simulink model "wlan_mac_hw"  (Simulink 7.8)
settings: Solver=ode45  StartTime=0.0  StopTime=200  RelTol=1e-3
PostLoadFcn:
  | wlan_mac_hw_init
InitFcn:
  | wlan_mac_hw_init
StartFcn:
  | wlan_mac_hw_init
values from neighbouring files (symbols this model uses):
  NB_CNTR_NAV = ceil(log2(MAX_NAV * 160))    [wlan_mac_hw_init.m]
  ticks_per_usec = 10    [wlan_mac_hw_init.m]
undefined symbols (not defined in the file or in its folder): gcbh, xlBlockLoadCallback, xlGetNormalizedPeriod
libraries: xbsIndex_r4 x788, xbsEDKLib_r4 x1
(part 3 of 6)

== system wlan_mac_hw/Idle for DIFS-EIFS ==
  note: IEEE 802.11-2012 9.3.4.2:
      | "medium is idle for a DIFS period...or an EIFS period if the immediately preceding medium-busy
      | event was caused by detection of a frame that was not received...with correct FCS".
      |
      | This logic reverts to DIFS on every new busy event, then
      | selects EIFS if there is an RX_END with errors.
  note: Counter stops after IDLE=1 longer than DIFS
      | IDLE_FOR_DIFS stays asserted until
      | the next medium busy event
  Bad Rx : Subsystem
  DIFS : xbsIndex_r4/Counter  cnt_type=Free Running  cnt_to=inf  operation=Up  start_count=0  cnt_by_val=1  arith_type=Unsigned  n_bits=NB_CNTR_DIFS  bin_pt=0  load_pin=off  rst=on  en=on  explicit_period=off  period=1  dbl_ovrd=off  use_behavioral_HDL=off  implementation=Fabric  block_type=counter
  Gateway Out{,4..6} (4 alike) : xbsIndex_r4/Gateway Out  inherit_from_input=off  hdl_port=off  timing_constraint=None  locs_specified=off  LOCs={}  UseAsDAC=off  DACChannel='1'  block_type=gatewayout
  IDLE for DIFS : Scope  NumInputPorts=7
      settings: YMin=-5~-5~-5~-5~-5~-5~-5  YMax=5~5~5~5~5~5~5  SaveName=ScopeData4
  Inverter : xbsIndex_r4/Inverter  en=off  latency=0  dbl_ovrd=off  block_type=inv
      settings: xl_area=[0 0 0 0 0 0 0]  block_version=VER_STRING_GOES_HERE
  Logical1 : xbsIndex_r4/Logical  logical_function=AND  inputs=2  en=off  latency=0  precision=Full  arith_type=Unsigned  n_bits=16  bin_pt=0  align_bp=on  dbl_ovrd=off  block_type=logical
  Logical2 : xbsIndex_r4/Logical  logical_function=OR  inputs=2  en=off  latency=0  precision=Full  arith_type=Unsigned  n_bits=8  bin_pt=2  align_bp=on  dbl_ovrd=off  block_type=logical
      settings: xl_area=[1 0 0 1 0 0 0]  block_version=VER_STRING_GOES_HERE
  Logical5 : xbsIndex_r4/Logical  logical_function=OR  inputs=3  en=off  latency=0  precision=Full  arith_type=Unsigned  n_bits=16  bin_pt=0  align_bp=on  dbl_ovrd=off  block_type=logical
  Mux : xbsIndex_r4/Mux  inputs=2  en=off  latency=0  precision=Full  arith_type=Unsigned  n_bits=16  bin_pt=14  quantization=Truncate  overflow=Wrap  dbl_ovrd=off  block_type=mux
  Mux1 : xbsIndex_r4/Mux  inputs=2  en=off  latency=0  precision=Full  arith_type=Unsigned  n_bits=16  bin_pt=14  quantization=Truncate  overflow=Wrap  dbl_ovrd=off  block_type=mux
  Register{,1..3} (4 alike) : xbsIndex_r4/Register  init=0  rst=off  en=off  dbl_ovrd=off  block_type=register
  Relational1 : xbsIndex_r4/Relational  mode=a>=b  en=off  latency=0  dbl_ovrd=off  block_type=relational
  Relational3 : xbsIndex_r4/Relational  mode=a>=b  en=off  latency=0  dbl_ovrd=off  block_type=relational
  S-R Latch1 : Subsystem
  dbg_EIFS_sel : xbsIndex_r4/Gateway Out  inherit_from_input=off  hdl_port=on  timing_constraint=None  locs_specified=off  LOCs={}  UseAsDAC=off  DACChannel='1'  block_type=gatewayout
  dbg_Idle_for_difs : xbsIndex_r4/Gateway Out  inherit_from_input=off  hdl_port=on  timing_constraint=None  locs_specified=off  LOCs={}  UseAsDAC=off  DACChannel='1'  block_type=gatewayout
  Idle for DIFS : Outport
  Idle for TxDIFS : Outport  Port=2
  wires:
  Relational3/1 -> Idle for DIFS/1, Inverter/1, Logical5/1, Gateway Out6/1
  Mux/1 -> Relational3/2
  DIFS/1 -> Relational3/1, Relational1/1, Gateway Out5/1
  Logical2/1 -> DIFS/1, Gateway Out4/1
  Logical1/1 -> DIFS/2, Gateway Out/1
  [MEDIUM_IDLE] -> Logical1/1
  [reg_Interval_DIFS] -> Mux/2
  [reg_Interval_EIFS] -> Mux/3
  S-R Latch1/1(Q) -> Mux/1, Mux1/1, Register2/1
  Bad Rx/1(Rx) -> S-R Latch1/1(S)
  Logical5/1 -> S-R Latch1/2(R)
  [MEDIUM_BUSY] -> Logical5/2
  [reg_CalibTime_TxDIFS] -> Mux1/2
  [reg_Interval_EIFS] -> Mux1/3
  Mux1/1 -> Relational1/2
  Relational1/1 -> Idle for TxDIFS/1, Register/1
  Inverter/1 -> Logical1/2
  Gateway Out/1 -> IDLE for DIFS/1
  Gateway Out4/1 -> IDLE for DIFS/5
  Gateway Out5/1 -> IDLE for DIFS/6
  Gateway Out6/1 -> IDLE for DIFS/7
  [GLOBAL_RESET] -> Logical5/3
  [MEDIUM_BUSY] -> Logical2/2
  [GLOBAL_RESET] -> Logical2/1
  Register/1 -> Register1/1
  Register1/1 -> dbg_Idle_for_difs/1
  Register2/1 -> Register3/1
  Register3/1 -> dbg_EIFS_sel/1

== system wlan_mac_hw/NAV ==
  note: NAV counter runs at core clock rate. Duration
      | values are scaled up from usec to core clock
      | (DURATION * 160 in ref design)
      |
      | NAV counter runs independent of any
      | other state (PHY CS, Tx state, etc.)
  note: Only use DURATION values greater
      | than current NAV value
  note: TODO: add NAV reset post-RTS when no RXSTART occurs
      | within a programmed time
  BitsM:4 : xbsIndex_r4/Slice  nbits=NB_CNTR_NAV-4  boolean_output=off  mode=Upper Bit Location + Width  bit1=0  base1=MSB of Input  bit0=0  base0=LSB of Input  dbl_ovrd=off  block_type=slice
  Constant : xbsIndex_r4/Constant  const=0  gui_display_data_type=Fixed-point  arith_type=Unsigned  n_bits=1  bin_pt=0  preci_type=Single  exp_width=8  frac_width=24  explicit_period=off  period=1  equ=P=C  opselect=C  inp2=PCIN>>17  opr=+  inp1=P  carry=CIN  dbl_ovrd=off  block_type=constant
  Convert : xbsIndex_r4/Convert  gui_display_data_type=Fixed-point  arith_type=Unsigned  n_bits=NB_CNTR_NAV  bin_pt=0  float_type=Single  exp_bits=8  fraction_bits=24  quantization=Truncate  overflow=Wrap  en=off  latency=0  dbl_ovrd=off  pipeline=off  block_type=convert
  Gateway Out{,1..3} (4 alike) : xbsIndex_r4/Gateway Out  inherit_from_input=off  hdl_port=off  timing_constraint=None  locs_specified=off  LOCs={}  UseAsDAC=off  DACChannel='1'  block_type=gatewayout
  Inverter : xbsIndex_r4/Inverter  en=off  latency=0  dbl_ovrd=off  block_type=inv
      settings: xl_area=[0 0 0 0 0 0 0]  block_version=VER_STRING_GOES_HERE
  Inverter1 : xbsIndex_r4/Inverter  en=off  latency=0  dbl_ovrd=off  block_type=inv
      settings: xl_area=[0 0 0 0 0 0 0]  block_version=VER_STRING_GOES_HERE
  Logical1 : xbsIndex_r4/Logical  logical_function=AND  inputs=2  en=off  latency=0  precision=Full  arith_type=Unsigned  n_bits=16  bin_pt=0  align_bp=on  dbl_ovrd=off  block_type=logical
  Logical2 : xbsIndex_r4/Logical  logical_function=OR  inputs=2  en=off  latency=0  precision=Full  arith_type=Unsigned  n_bits=16  bin_pt=0  align_bp=on  dbl_ovrd=off  block_type=logical
  Logical3 : xbsIndex_r4/Logical  logical_function=AND  inputs=2  en=off  latency=0  precision=Full  arith_type=Unsigned  n_bits=16  bin_pt=0  align_bp=on  dbl_ovrd=off  block_type=logical
  Logical4 : xbsIndex_r4/Logical  logical_function=OR  inputs=2  en=off  latency=0  precision=Full  arith_type=Unsigned  n_bits=16  bin_pt=0  align_bp=on  dbl_ovrd=off  block_type=logical
  NAV : Scope  NumInputPorts=7
      settings: YMin=-5~-5~-5~-5~-5~-5~-5  YMax=5~5~5~5~5~5~5  SaveName=ScopeData3
  NAV Counter : xbsIndex_r4/Counter  cnt_type=Free Running  cnt_to=Inf  operation=Down  start_count=0  cnt_by_val=1  arith_type=Unsigned  n_bits=NB_CNTR_NAV  bin_pt=0  load_pin=on  rst=on  en=on  explicit_period=on  period=1  dbl_ovrd=off  use_behavioral_HDL=off  implementation=Fabric  block_type=counter
  New Duration : Subsystem
  Register : xbsIndex_r4/Register  init=0  rst=off  en=off  dbl_ovrd=off  block_type=register
  Register1 : xbsIndex_r4/Register  init=0  rst=off  en=off  dbl_ovrd=off  block_type=register
  Relational1 : xbsIndex_r4/Relational  mode=a<b  en=off  latency=0  dbl_ovrd=off  block_type=relational
  Relational2 : xbsIndex_r4/Relational  mode=a>b  en=off  latency=0  dbl_ovrd=off  block_type=relational
  dbg_NAV_Active : xbsIndex_r4/Gateway Out  inherit_from_input=off  hdl_port=on  timing_constraint=None  locs_specified=off  LOCs={}  UseAsDAC=off  DACChannel='1'  block_type=gatewayout
  NAV Busy : Outport
  tag scope: NAV_VALUE_100NSEC=global, NAV_Zero=global
  wires:
  Logical1/1 -> NAV Counter/1, Logical2/1, Gateway Out2/1
  New Duration/2(Valid) -> Logical1/2
  NAV Counter/1 -> Relational2/1, Relational1/1, BitsM:4/1, Gateway Out3/1
  Logical4/1 -> NAV Counter/3
  Constant/1 -> Relational2/2
  Relational2/1 -> Gateway Out/1, Logical2/2, Logical3/2
  New Duration/1(Duration) -> Relational1/2, Convert/1, Gateway Out1/1
  Relational1/1 -> Logical1/1
  Convert/1 -> NAV Counter/2
  Gateway Out/1 -> NAV/1
  Gateway Out1/1 -> NAV/2
  Gateway Out2/1 -> NAV/3
  Gateway Out3/1 -> NAV/4
  Logical2/1 -> NAV Counter/4
  Logical3/1 -> NAV Busy/1, Register/1, Inverter1/1
  [reg_Disable_NAV] -> Inverter/1
  Inverter/1 -> Logical3/1
  Register/1 -> Register1/1
  Register1/1 -> dbg_NAV_Active/1
  BitsM:4/1 -> [NAV_VALUE_100NSEC]
  [GLOBAL_RESET] -> Logical4/1
  [reg_Force_Reset_NAV] -> Logical4/2
  Inverter1/1 -> [NAV_Zero]

== system wlan_mac_hw/PHY I/O ==
  note: FCS_Good is valid starting when
      | data_done = 1 and stays valid through
      | rx_end = 1
  note: RX_ACTIVE status bit needs delay, so MPDU Tx FSM has time to declare TX_DONE
      |   due to RX_STARTED before the MAC code is notified that RX_STARTED
  Delay : xbsIndex_r4/Delay  rst=off  infoeditControl=Selection of Reset will increase slice count due to use of real FFs and instead of SRLs  en=off  latency=3  dbl_ovrd=off  reg_retiming=off  block_type=delay
  Logical1 : xbsIndex_r4/Logical  logical_function=OR  inputs=2  en=off  latency=0  precision=Full  arith_type=Unsigned  n_bits=8  bin_pt=2  align_bp=on  dbl_ovrd=off  block_type=logical
      settings: xl_area=[1 0 0 1 0 0 0]  block_version=VER_STRING_GOES_HERE
  Logical4 : xbsIndex_r4/Logical  logical_function=OR  inputs=2  en=off  latency=0  precision=Full  arith_type=Unsigned  n_bits=8  bin_pt=2  align_bp=on  dbl_ovrd=off  block_type=logical
      settings: xl_area=[1 0 0 1 0 0 0]  block_version=VER_STRING_GOES_HERE
  PHY Rx Ports : Subsystem
  PHY Tx Ports : Subsystem
  Register3 : xbsIndex_r4/Register  init=0  rst=on  en=on  dbl_ovrd=off  block_type=register
  S-R Latch2 : Subsystem
  S-R Latch3 : Subsystem
  tag scope: Status_Rx_FCS_Good=global, Status_Rx_PHY_Active=global, Status_Tx_PHY_Active=global
  wires:
  [PHY_TX_START_CONFIRM] -> S-R Latch2/1(S)
  Logical1/1 -> S-R Latch2/2(R)
  [PHY_TX_END_CONFIRM] -> Logical1/1
  [GLOBAL_RESET] -> Logical1/2
  S-R Latch2/1(Q) -> [Status_Tx_PHY_Active]
  [PHY_RX_START_IND] -> S-R Latch3/1(S)
  Logical4/1 -> S-R Latch3/2(R)
  [PHY_RX_END_IND] -> Logical4/1
  [GLOBAL_RESET] -> Logical4/2
  S-R Latch3/1(Q) -> Delay/1
  [PHY_RX_FCS_GOOD_IND] -> Register3/1
  Register3/1 -> [Status_Rx_FCS_Good]
  [PHY_RX_DATA_DONE_IND] -> Register3/3
  [PHY_RX_START_IND] -> Register3/2
  Delay/1 -> [Status_Rx_PHY_Active]

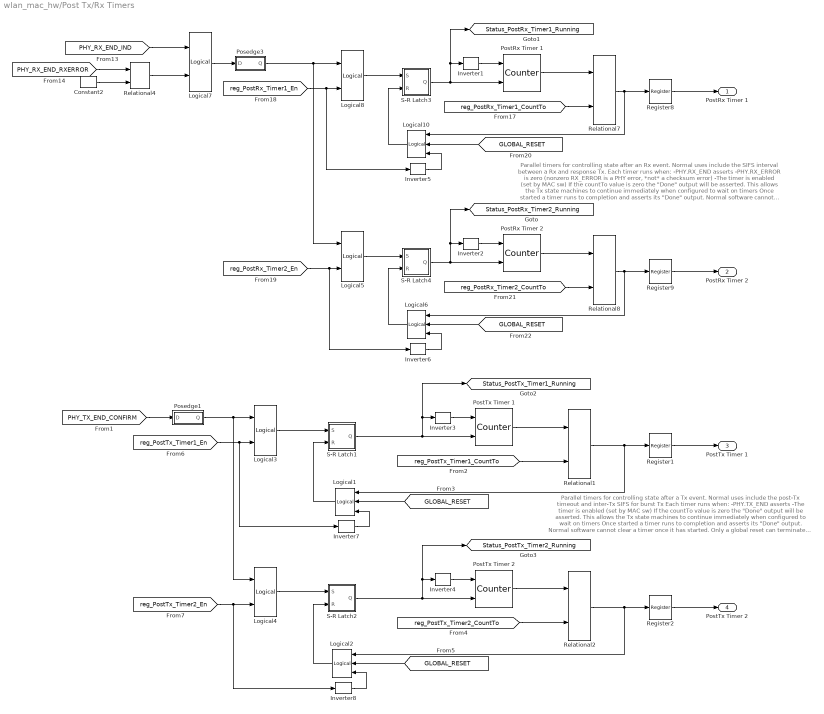
== system wlan_mac_hw/Post Tx/Rx Timers ==
  note: Parallel timers for controlling state after an Rx event. Normal uses include the SIFS interval
      |  between a Rx and response Tx.
      |
      | Each timer runs when:
      | -PHY.RX_END asserts
      | -PHY.RX_ERROR is zero (nonzero RX_ERROR is a PHY error, *not* a checksum error)
      | -The timer is enabled (set by MAC sw)
      |
      | If the countTo value is zero the "Done" output will be asserted. This allows the Tx state
      |  machines to continue immediately when configured to wait on timers
      |
      | Once started a timer runs to completion and asserts its "Done" output. Normal software
      | cannot clear a timer once it has started. Only a global reset can terminate a timer before
      | it completes. Downstream logic using the "Done" signal should apply its own conditions
      | when deciding whether to act on the timer expiring.
  note: Parallel timers for controlling state after a Tx event. Normal uses include the post-Tx
      | timeout and inter-Tx SIFS for burst Tx
      |
      | Each timer runs when:
      | -PHY.TX_END asserts
      | -The timer is enabled (set by MAC sw)
      |
      | If the countTo value is zero the "Done" output will be asserted. This allows the Tx state
      |  machines to continue immediately when configured to wait on timers
      |
      | Once started a timer runs to completion and asserts its "Done" output. Normal software
      | cannot clear a timer once it has started. Only a global reset can terminate a timer before
      | it completes. Downstream logic using the "Done" signal should apply its own conditions
      | when deciding whether to act on the timer expiring.
  Constant2 : xbsIndex_r4/Constant  const=0  gui_display_data_type=Fixed-point  arith_type=Unsigned  n_bits=1  bin_pt=0  preci_type=Single  exp_width=8  frac_width=24  explicit_period=off  period=1  equ=P=C  opselect=C  inp2=PCIN>>17  opr=+  inp1=P  carry=CIN  dbl_ovrd=off  block_type=constant
  Inverter{1..8} (8 alike) : xbsIndex_r4/Inverter  en=off  latency=0  dbl_ovrd=off  block_type=inv
      settings: xl_area=[0 0 0 0 0 0 0]  block_version=VER_STRING_GOES_HERE
  Logical{1..2,6,10} (4 alike) : xbsIndex_r4/Logical  logical_function=OR  inputs=3  en=off  latency=0  precision=Full  arith_type=Unsigned  n_bits=8  bin_pt=2  align_bp=on  dbl_ovrd=off  block_type=logical
      settings: xl_area=[1 0 0 1 0 0 0]  block_version=VER_STRING_GOES_HERE
  Logical{3..5,7..8} (5 alike) : xbsIndex_r4/Logical  logical_function=AND  inputs=2  en=off  latency=0  precision=Full  arith_type=Unsigned  n_bits=16  bin_pt=0  align_bp=on  dbl_ovrd=off  block_type=logical
  Posedge1 : Subsystem
  Posedge3 : Subsystem
  PostRx Timer 1 : xbsIndex_r4/Counter  cnt_type=Free Running  cnt_to=1  operation=Up  start_count=0  cnt_by_val=1  arith_type=Unsigned  n_bits=NB_CNTR_POSTRX  bin_pt=0  load_pin=off  rst=on  en=on  explicit_period=off  period=1  dbl_ovrd=off  use_behavioral_HDL=off  implementation=Fabric  block_type=counter
  PostRx Timer 2 : xbsIndex_r4/Counter  cnt_type=Free Running  cnt_to=1  operation=Up  start_count=0  cnt_by_val=1  arith_type=Unsigned  n_bits=NB_CNTR_POSTRX  bin_pt=0  load_pin=off  rst=on  en=on  explicit_period=off  period=1  dbl_ovrd=off  use_behavioral_HDL=off  implementation=Fabric  block_type=counter
  PostTx Timer 1 : xbsIndex_r4/Counter  cnt_type=Free Running  cnt_to=1  operation=Up  start_count=0  cnt_by_val=1  arith_type=Unsigned  n_bits=NB_CNTR_POSTRX  bin_pt=0  load_pin=off  rst=on  en=on  explicit_period=off  period=1  dbl_ovrd=off  use_behavioral_HDL=off  implementation=Fabric  block_type=counter
  PostTx Timer 2 : xbsIndex_r4/Counter  cnt_type=Free Running  cnt_to=1  operation=Up  start_count=0  cnt_by_val=1  arith_type=Unsigned  n_bits=NB_CNTR_POSTRX  bin_pt=0  load_pin=off  rst=on  en=on  explicit_period=off  period=1  dbl_ovrd=off  use_behavioral_HDL=off  implementation=Fabric  block_type=counter
  Register{1..2,8..9} (4 alike) : xbsIndex_r4/Register  init=0  rst=off  en=off  dbl_ovrd=off  block_type=register
      settings: xl_area=[1 1 0 0 0 0 0]  block_version=VER_STRING_GOES_HERE
  Relational{1..2,7..8} (4 alike) : xbsIndex_r4/Relational  mode=a>=b  en=off  latency=0  dbl_ovrd=off  block_type=relational
  Relational4 : xbsIndex_r4/Relational  mode=a=b  en=off  latency=0  dbl_ovrd=off  block_type=relational
  S-R Latch1 : Subsystem
  S-R Latch2 : Subsystem
  S-R Latch3 : Subsystem
  S-R Latch4 : Subsystem
  " PostRx Timer 1" : Outport
  " PostRx Timer 2" : Outport  Port=2
  " PostTx Timer 1" : Outport  Port=3
  " PostTx Timer 2" : Outport  Port=4
  tag scope: Status_PostRx_Timer1_Running=global, Status_PostRx_Timer2_Running=global, Status_PostTx_Timer1_Running=global, Status_PostTx_Timer2_Running=global
  wires:
  [PHY_RX_END_RXERROR] -> Relational4/1
  Constant2/1 -> Relational4/2
  [PHY_RX_END_IND] -> Logical7/1
  Relational4/1 -> Logical7/2
  Logical7/1 -> Posedge3/1(D)
  Posedge3/1(Q) -> Logical8/1, Logical5/1
  Logical8/1 -> S-R Latch3/1(S)
  S-R Latch3/1(Q) -> PostRx Timer 1/2, Inverter1/1, [Status_PostRx_Timer1_Running]
  Inverter1/1 -> PostRx Timer 1/1
  PostRx Timer 1/1 -> Relational7/1
  [reg_PostRx_Timer1_CountTo] -> Relational7/2
  [reg_PostRx_Timer1_En] -> Logical8/2, Inverter5/1
  Relational7/1 -> Register8/1, Logical10/1
  Register8/1 -> " PostRx Timer 1"/1
  Logical10/1 -> S-R Latch3/2(R)
  [GLOBAL_RESET] -> Logical10/2
  Logical5/1 -> S-R Latch4/1(S)
  S-R Latch4/1(Q) -> PostRx Timer 2/2, Inverter2/1, [Status_PostRx_Timer2_Running]
  Inverter2/1 -> PostRx Timer 2/1
  PostRx Timer 2/1 -> Relational8/1
  [reg_PostRx_Timer2_CountTo] -> Relational8/2
  Relational8/1 -> Register9/1, Logical6/1
  Logical6/1 -> S-R Latch4/2(R)
  [GLOBAL_RESET] -> Logical6/2
  Register9/1 -> " PostRx Timer 2"/1
  [PHY_TX_END_CONFIRM] -> Posedge1/1(D)
  Inverter3/1 -> PostTx Timer 1/1
  S-R Latch1/1(Q) -> PostTx Timer 1/2, Inverter3/1, [Status_PostTx_Timer1_Running]
  PostTx Timer 1/1 -> Relational1/1
  [reg_PostTx_Timer1_CountTo] -> Relational1/2
  [GLOBAL_RESET] -> Logical1/2
  Logical1/1 -> S-R Latch1/2(R)
  Relational1/1 -> Register1/1, Logical1/1
  Register1/1 -> " PostTx Timer 1"/1
  Inverter4/1 -> PostTx Timer 2/1
  S-R Latch2/1(Q) -> PostTx Timer 2/2, Inverter4/1, [Status_PostTx_Timer2_Running]
  PostTx Timer 2/1 -> Relational2/1
  [reg_PostTx_Timer2_CountTo] -> Relational2/2
  [GLOBAL_RESET] -> Logical2/2
  Logical2/1 -> S-R Latch2/2(R)
  Relational2/1 -> Register2/1, Logical2/1
  Register2/1 -> " PostTx Timer 2"/1
  Logical3/1 -> S-R Latch1/1(S)
  Posedge1/1(Q) -> Logical3/1, Logical4/1
  [reg_PostTx_Timer1_En] -> Logical3/2, Inverter7/1
  [reg_PostTx_Timer2_En] -> Logical4/2, Inverter8/1
  Logical4/1 -> S-R Latch2/1(S)
  [reg_PostRx_Timer2_En] -> Logical5/2, Inverter6/1
  Inverter5/1 -> Logical10/3
  Inverter6/1 -> Logical6/3
  Inverter7/1 -> Logical1/3
  Inverter8/1 -> Logical2/3

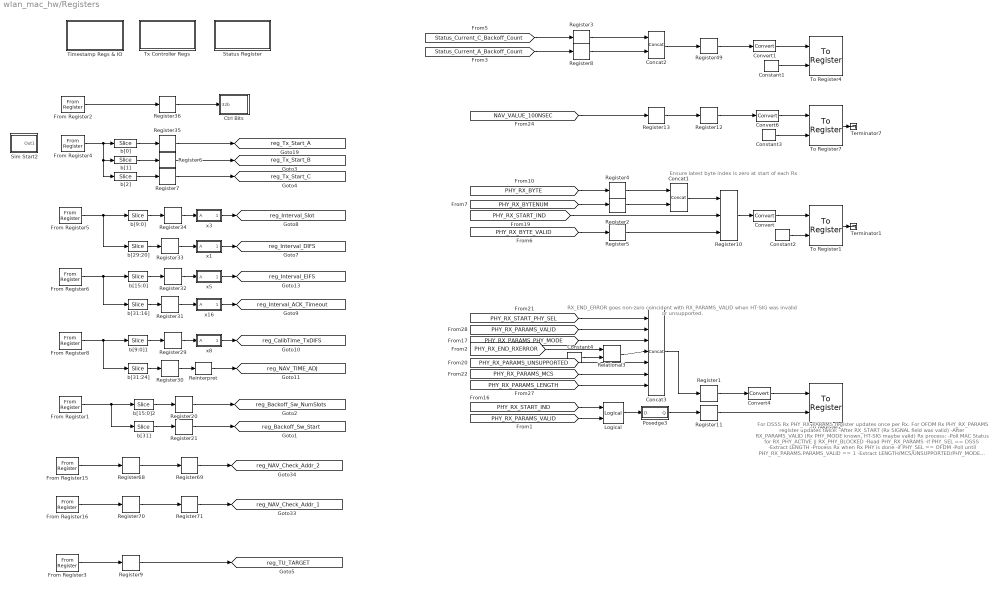
== system wlan_mac_hw/Registers ==
  note: Ensure latest byte index is zero
      | at start of each Rx
  note: For DSSS Rx PHY_RX_PARAMS register updates once per Rx.
      | For OFDM Rx PHY_RX_PARAMS register updates twice:
      |   -After RX_START (Rx SIGNAL field was valid)
      |   -After RX_PARAMS_VALID (Rx PHY_MODE known, HT-SIG maybe valid)
      |
      | Rx process:
      | -Poll MAC Status for RX_PHY_ACTIVE || RX_PHY_BLOCKED
      | -Read PHY_RX_PARAMS
      |   -if PHY_SEL == DSSS
      |     -Extract LENGTH
      |     -Process Rx when Rx PHY is done
      |   -if PHY_SEL == OFDM
      |     -Poll until PHY_RX_PARAMS.PARAMS_VALID == 1
      |      -Extract LENGTH/MCS/UNSUPPORTED/PHY_MODE
      |      -Process Rx when Rx PHY is done
  note: RX_END_ERROR goes non-zero coincident with
      | RX_PARAMS_VALID when HT-SIG was invalid
      | or unsupported.
  " b[15:0]" : xbsIndex_r4/Slice  nbits=16  boolean_output=off  mode=Lower Bit Location + Width  bit1=0  base1=MSB of Input  bit0=0  base0=LSB of Input  dbl_ovrd=off  block_type=slice
      settings: block_version=VER_STRING_GOES_HERE
  " b[15:0]2" : xbsIndex_r4/Slice  nbits=16  boolean_output=off  mode=Lower Bit Location + Width  bit1=0  base1=MSB of Input  bit0=0  base0=LSB of Input  dbl_ovrd=off  block_type=slice
      settings: block_version=VER_STRING_GOES_HERE
  " b[29:20]" : xbsIndex_r4/Slice  nbits=10  boolean_output=off  mode=Lower Bit Location + Width  bit1=0  base1=MSB of Input  bit0=20  base0=LSB of Input  dbl_ovrd=off  block_type=slice
      settings: block_version=VER_STRING_GOES_HERE
  " b[31:16]" : xbsIndex_r4/Slice  nbits=16  boolean_output=off  mode=Lower Bit Location + Width  bit1=0  base1=MSB of Input  bit0=16  base0=LSB of Input  dbl_ovrd=off  block_type=slice
      settings: block_version=VER_STRING_GOES_HERE
  " b[31:24]" : xbsIndex_r4/Slice  nbits=8  boolean_output=off  mode=Lower Bit Location + Width  bit1=0  base1=MSB of Input  bit0=24  base0=LSB of Input  dbl_ovrd=off  block_type=slice
      settings: block_version=VER_STRING_GOES_HERE
  " b[31]" : xbsIndex_r4/Slice  nbits=1  boolean_output=on  mode=Lower Bit Location + Width  bit1=0  base1=MSB of Input  bit0=31  base0=LSB of Input  dbl_ovrd=off  block_type=slice
      settings: block_version=VER_STRING_GOES_HERE
  " b[9:0]" : xbsIndex_r4/Slice  nbits=10  boolean_output=off  mode=Lower Bit Location + Width  bit1=0  base1=MSB of Input  bit0=0  base0=LSB of Input  dbl_ovrd=off  block_type=slice
      settings: block_version=VER_STRING_GOES_HERE
  " b[9:0]1" : xbsIndex_r4/Slice  nbits=10  boolean_output=off  mode=Lower Bit Location + Width  bit1=0  base1=MSB of Input  bit0=0  base0=LSB of Input  dbl_ovrd=off  block_type=slice
      settings: block_version=VER_STRING_GOES_HERE
  Concat1 : xbsIndex_r4/Concat  num_inputs=2  dbl_ovrd=off  block_type=concat
      settings: block_version=8.2.02
  Concat2 : xbsIndex_r4/Concat  num_inputs=2  dbl_ovrd=off  block_type=concat
      settings: block_version=8.2.02
  Concat3 : xbsIndex_r4/Concat  num_inputs=7  dbl_ovrd=off  block_type=concat
      settings: block_version=8.2.02
  Constant1 : xbsIndex_r4/Constant  const=1  gui_display_data_type=Boolean  arith_type=Boolean  n_bits=30  bin_pt=0  preci_type=Single  exp_width=8  frac_width=24  explicit_period=on  period=1  equ=P=C  opselect=C  inp2=PCIN>>17  opr=+  inp1=P  carry=CIN  dbl_ovrd=off  block_type=constant
  Constant2 : xbsIndex_r4/Constant  const=1  gui_display_data_type=Boolean  arith_type=Boolean  n_bits=30  bin_pt=0  preci_type=Single  exp_width=8  frac_width=24  explicit_period=on  period=1  equ=P=C  opselect=C  inp2=PCIN>>17  opr=+  inp1=P  carry=CIN  dbl_ovrd=off  block_type=constant
  Constant3 : xbsIndex_r4/Constant  const=1  gui_display_data_type=Boolean  arith_type=Boolean  n_bits=30  bin_pt=0  preci_type=Single  exp_width=8  frac_width=24  explicit_period=on  period=1  equ=P=C  opselect=C  inp2=PCIN>>17  opr=+  inp1=P  carry=CIN  dbl_ovrd=off  block_type=constant
  Constant4 : xbsIndex_r4/Constant  const=0  gui_display_data_type=Fixed-point  arith_type=Unsigned  n_bits=1  bin_pt=0  preci_type=Single  exp_width=8  frac_width=24  explicit_period=off  period=1  equ=P=C  opselect=C  inp2=PCIN>>17  opr=+  inp1=P  carry=CIN  dbl_ovrd=off  block_type=constant
  Convert{,1,4,6} (4 alike) : xbsIndex_r4/Convert  gui_display_data_type=Fixed-point  arith_type=Unsigned  n_bits=32  bin_pt=0  float_type=Single  exp_bits=8  fraction_bits=24  quantization=Truncate  overflow=Wrap  en=off  latency=0  dbl_ovrd=off  pipeline=off  block_type=convert
  Ctrl Bits : Subsystem
  From Register1 : xbsIndex_r4/From Register  shared_memory_name='BACKOFF_CTRL'  init=REG_MAC_Backoff_Control  period=1  ownership=Locally owned and initialized  gui_display_data_type=Fixed-point  arith_type=Unsigned  n_bits=32  bin_pt=0  preci_type=Single  dbl_ovrd=off  block_type=fromreg
      settings: AttributesFormatString=<< %<shared_memory_name> >>  infoedit="Register block that reads data to a shared memory register.  Delay of one sample period."
  From Register15 : xbsIndex_r4/From Register  shared_memory_name='NAV_MATCH_ADDR_2'  init=REG_NAV_Match_Addr_2  period=1  ownership=Locally owned and initialized  gui_display_data_type=Fixed-point  arith_type=Unsigned  n_bits=32  bin_pt=0  preci_type=Single  dbl_ovrd=off  block_type=fromreg
      settings: AttributesFormatString=<< %<shared_memory_name> >>  infoedit="Register block that reads data to a shared memory register.  Delay of one sample period."
  From Register16 : xbsIndex_r4/From Register  shared_memory_name='NAV_MATCH_ADDR_1'  init=REG_NAV_Match_Addr_1  period=1  ownership=Locally owned and initialized  gui_display_data_type=Fixed-point  arith_type=Unsigned  n_bits=32  bin_pt=0  preci_type=Single  dbl_ovrd=off  block_type=fromreg
      settings: AttributesFormatString=<< %<shared_memory_name> >>  infoedit="Register block that reads data to a shared memory register.  Delay of one sample period."
  From Register2 : xbsIndex_r4/From Register  shared_memory_name='Control'  init=REG_MAC_Control  period=1  ownership=Locally owned and initialized  gui_display_data_type=Fixed-point  arith_type=Unsigned  n_bits=32  bin_pt=0  preci_type=Single  dbl_ovrd=off  block_type=fromreg
      settings: AttributesFormatString=<< %<shared_memory_name> >>  infoedit="Register block that reads data to a shared memory register.  Delay of one sample period."
  From Register3 : xbsIndex_r4/From Register  shared_memory_name='TU_TARGET'  init=2^32-1  period=1  ownership=Locally owned and initialized  gui_display_data_type=Fixed-point  arith_type=Unsigned  n_bits=32  bin_pt=0  preci_type=Single  dbl_ovrd=off  block_type=fromreg
      settings: AttributesFormatString=<< %<shared_memory_name> >>  infoedit="Register block that reads data to a shared memory register.  Delay of one sample period."
  From Register4 : xbsIndex_r4/From Register  shared_memory_name='TX_START'  init=0  period=1  ownership=Locally owned and initialized  gui_display_data_type=Fixed-point  arith_type=Unsigned  n_bits=32  bin_pt=0  preci_type=Single  dbl_ovrd=off  block_type=fromreg
      settings: AttributesFormatString=<< %<shared_memory_name> >>  infoedit="Register block that reads data to a shared memory register.  Delay of one sample period."
  From Register5 : xbsIndex_r4/From Register  shared_memory_name='IFS_INTERVALS1'  init=REG_MAC_Intervals_1  period=1  ownership=Locally owned and initialized  gui_display_data_type=Fixed-point  arith_type=Unsigned  n_bits=32  bin_pt=0  preci_type=Single  dbl_ovrd=off  block_type=fromreg
      settings: AttributesFormatString=<< %<shared_memory_name> >>  infoedit="Register block that reads data to a shared memory register.  Delay of one sample period."
  From Register6 : xbsIndex_r4/From Register  shared_memory_name='IFS_INTERVALS2'  init=REG_MAC_Intervals_2  period=1  ownership=Locally owned and initialized  gui_display_data_type=Fixed-point  arith_type=Unsigned  n_bits=32  bin_pt=0  preci_type=Single  dbl_ovrd=off  block_type=fromreg
      settings: AttributesFormatString=<< %<shared_memory_name> >>  infoedit="Register block that reads data to a shared memory register.  Delay of one sample period."
  From Register8 : xbsIndex_r4/From Register  shared_memory_name='CALIB_TIMES'  init=REG_MAC_Calib_Times  period=1  ownership=Locally owned and initialized  gui_display_data_type=Fixed-point  arith_type=Unsigned  n_bits=32  bin_pt=0  preci_type=Single  dbl_ovrd=off  block_type=fromreg
      settings: AttributesFormatString=<< %<shared_memory_name> >>  infoedit="Register block that reads data to a shared memory register.  Delay of one sample period."
  Logical : xbsIndex_r4/Logical  logical_function=OR  inputs=2  en=off  latency=0  precision=Full  arith_type=Unsigned  n_bits=16  bin_pt=0  align_bp=on  dbl_ovrd=off  block_type=logical
  Posedge3 : Subsystem
  Register{1..9,11..13,20..21,29..36,49,68..71} (27 alike) : xbsIndex_r4/Register  init=0  rst=off  en=off  dbl_ovrd=off  block_type=register
  Register10 : xbsIndex_r4/Register  init=0  rst=on  en=on  dbl_ovrd=off  block_type=register
  Reinterpret : xbsIndex_r4/Reinterpret  force_arith_type=on  arith_type="Signed  (2's comp)"  force_bin_pt=off  bin_pt=0  block_type=reinterpret
  Relational3 : xbsIndex_r4/Relational  mode=a!=b  en=off  latency=0  dbl_ovrd=off  block_type=relational
  Sim Start2 : Subsystem
  Status Register : Subsystem
  Terminator1 : Terminator
  Terminator7 : Terminator
  Timestamp Regs & IO : Subsystem
  To Register1 : xbsIndex_r4/To Register  shared_memory_name='LATEST_RX_BYTE'  init=0  ownership=Locally owned and initialized  explicit_data_type=on  gui_display_data_type=Fixed-point  arith_type=Unsigned  n_bits=32  bin_pt=0  preci_type=Single  dbl_ovrd=off  block_type=toreg
      settings: AttributesFormatString=<< %<shared_memory_name> >>  infoedit="Register block that writes data to a shared memory register.  Delay of one sample period."
  To Register2 : xbsIndex_r4/To Register  shared_memory_name='PHY_RX_PARAMS'  init=0  ownership=Locally owned and initialized  explicit_data_type=on  gui_display_data_type=Fixed-point  arith_type=Unsigned  n_bits=32  bin_pt=0  preci_type=Single  dbl_ovrd=off  block_type=toreg
      settings: AttributesFormatString=<< %<shared_memory_name> >>  infoedit="Register block that writes data to a shared memory register.  Delay of one sample period."
  To Register4 : xbsIndex_r4/To Register  shared_memory_name='BACKOFF_COUNTERS'  init=0  ownership=Locally owned and initialized  explicit_data_type=on  gui_display_data_type=Fixed-point  arith_type=Unsigned  n_bits=32  bin_pt=0  preci_type=Single  dbl_ovrd=off  block_type=toreg
      settings: AttributesFormatString=<< %<shared_memory_name> >>  infoedit="Register block that writes data to a shared memory register.  Delay of one sample period."
  To Register7 : xbsIndex_r4/To Register  shared_memory_name='NAV_VALUE'  init=0  ownership=Locally owned and initialized  explicit_data_type=on  gui_display_data_type=Fixed-point  arith_type=Unsigned  n_bits=32  bin_pt=0  preci_type=Single  dbl_ovrd=off  block_type=toreg
      settings: AttributesFormatString=<< %<shared_memory_name> >>  infoedit="Register block that writes data to a shared memory register.  Delay of one sample period."
  Tx Controller Regs : Subsystem
  "b[0] " : xbsIndex_r4/Slice  nbits=1  boolean_output=on  mode=Lower Bit Location + Width  bit1=0  base1=MSB of Input  bit0=0  base0=LSB of Input  dbl_ovrd=off  block_type=slice
      settings: block_version=VER_STRING_GOES_HERE
  b[1] : xbsIndex_r4/Slice  nbits=1  boolean_output=on  mode=Lower Bit Location + Width  bit1=0  base1=MSB of Input  bit0=1  base0=LSB of Input  dbl_ovrd=off  block_type=slice
      settings: block_version=VER_STRING_GOES_HERE
  b[2] : xbsIndex_r4/Slice  nbits=1  boolean_output=on  mode=Lower Bit Location + Width  bit1=0  base1=MSB of Input  bit0=2  base0=LSB of Input  dbl_ovrd=off  block_type=slice
      settings: block_version=VER_STRING_GOES_HERE
  x1 : Subsystem
  x16 : Subsystem
  x3 : Subsystem
  x5 : Subsystem
  x8 : Subsystem
  tag scope: reg_Backoff_Sw_NumSlots=global, reg_Backoff_Sw_Start=global, reg_CalibTime_TxDIFS=global, reg_Interval_ACK_Timeout=global, reg_Interval_DIFS=global, reg_Interval_EIFS=global, reg_Interval_Slot=global, reg_NAV_Check_Addr_1=global, reg_NAV_Check_Addr_2=global, reg_NAV_TIME_ADJ=global, reg_TU_TARGET=global, reg_Tx_Start_A=global, reg_Tx_Start_B=global, reg_Tx_Start_C=global
  wires:
  From Register2/1 -> Register36/1
  x16/1(Ax16) -> [reg_Interval_ACK_Timeout]
  x1/1(Ax16) -> [reg_Interval_DIFS]
  x3/1(Ax16) -> [reg_Interval_Slot]
  x5/1(Ax16) -> [reg_Interval_EIFS]
  "b[0] "/1 -> Register35/1
  From Register5/1 -> " b[9:0]"/1, " b[29:20]"/1
  From Register6/1 -> " b[15:0]"/1, " b[31:16]"/1
  " b[9:0]"/1 -> Register34/1
  " b[29:20]"/1 -> Register33/1
  " b[15:0]"/1 -> Register32/1
  " b[31:16]"/1 -> Register31/1
  x8/1(Ax16) -> [reg_CalibTime_TxDIFS]
  From Register8/1 -> " b[9:0]1"/1, " b[31:24]"/1
  " b[9:0]1"/1 -> Register29/1
  " b[31:24]"/1 -> Register30/1
  From Register1/1 -> " b[15:0]2"/1, " b[31]"/1
  " b[15:0]2"/1 -> Register20/1
  " b[31]"/1 -> Register21/1
  To Register1/1 -> Terminator1/1
  [PHY_RX_BYTE_VALID] -> Register5/1
  [PHY_RX_BYTENUM] -> Register2/1
  Register2/1 -> Concat1/2
  Register4/1 -> Concat1/1
  Register5/1 -> Register10/3
  [PHY_RX_BYTE] -> Register4/1
  From Register4/1 -> "b[0] "/1, b[1]/1, b[2]/1
  Concat1/1 -> Register10/1
  [PHY_RX_START_IND] -> Logical/1
  Register10/1 -> Convert/1
  Convert/1 -> To Register1/1
  Constant2/1 -> To Register1/2
  [PHY_RX_START_IND] -> Register10/2
  Reinterpret/1 -> [reg_NAV_TIME_ADJ]
  To Register7/1 -> Terminator7/1
  [NAV_VALUE_100NSEC] -> Register13/1
  Convert6/1 -> To Register7/1
  Register12/1 -> Convert6/1
  Register13/1 -> Register12/1
  Constant3/1 -> To Register7/2
  Register20/1 -> [reg_Backoff_Sw_NumSlots]
  Register21/1 -> [reg_Backoff_Sw_Start]
  Register29/1 -> x8/1(A)
  Register30/1 -> Reinterpret/1
  Register31/1 -> x16/1(A)
  Register32/1 -> x5/1(A)
  Register33/1 -> x1/1(A)
  Register34/1 -> x3/1(A)
  Register35/1 -> [reg_Tx_Start_A]
  Register36/1 -> Ctrl Bits/1(32b)
  From Register15/1 -> Register68/1
  Register68/1 -> Register69/1
  Register69/1 -> [reg_NAV_Check_Addr_2]
  From Register16/1 -> Register70/1
  Register70/1 -> Register71/1
  Register71/1 -> [reg_NAV_Check_Addr_1]
  Posedge3/1(Q) -> Register11/1
  Register1/1 -> Convert4/1
  Register11/1 -> To Register2/2
  [PHY_RX_PARAMS_VALID] -> Logical/2
  Logical/1 -> Posedge3/1(D)
  b[1]/1 -> Register6/1
  Register6/1 -> [reg_Tx_Start_B]
  Concat3/1 -> Register1/1
  Convert4/1 -> To Register2/1
  Register49/1 -> Convert1/1
  Constant1/1 -> To Register4/2
  Convert1/1 -> To Register4/1
  [PHY_RX_PARAMS_LENGTH] -> Concat3/7
  [PHY_RX_PARAMS_UNSUPPORTED] -> Concat3/5
  [PHY_RX_PARAMS_MCS] -> Concat3/6
  Constant4/1 -> Relational3/2
  [PHY_RX_END_RXERROR] -> Relational3/1
  Relational3/1 -> Concat3/4
  [PHY_RX_START_PHY_SEL] -> Concat3/1
  [PHY_RX_PARAMS_VALID] -> Concat3/2
  [PHY_RX_PARAMS_PHY_MODE] -> Concat3/3
  b[2]/1 -> Register7/1
  Register7/1 -> [reg_Tx_Start_C]
  Concat2/1 -> Register49/1
  Register3/1 -> Concat2/1
  [Status_Current_C_Backoff_Count] -> Register3/1
  Register8/1 -> Concat2/2
  [Status_Current_A_Backoff_Count] -> Register8/1
  From Register3/1 -> Register9/1
  Register9/1 -> [reg_TU_TARGET]

== system wlan_mac_hw/Slot Time ==
  note: Counter starts over if it is disabled
  Gateway Out : xbsIndex_r4/Gateway Out  inherit_from_input=off  hdl_port=off  timing_constraint=None  locs_specified=off  LOCs={}  UseAsDAC=off  DACChannel='1'  block_type=gatewayout
  Gateway Out1 : xbsIndex_r4/Gateway Out  inherit_from_input=off  hdl_port=off  timing_constraint=None  locs_specified=off  LOCs={}  UseAsDAC=off  DACChannel='1'  block_type=gatewayout
  Gateway Out3 : xbsIndex_r4/Gateway Out  inherit_from_input=off  hdl_port=off  timing_constraint=None  locs_specified=off  LOCs={}  UseAsDAC=off  DACChannel='1'  block_type=gatewayout
  Inverter : xbsIndex_r4/Inverter  en=off  latency=0  dbl_ovrd=off  block_type=inv
      settings: xl_area=[0 0 0 0 0 0 0]  block_version=VER_STRING_GOES_HERE
  Logical1 : xbsIndex_r4/Logical  logical_function=OR  inputs=2  en=off  latency=0  precision=Full  arith_type=Unsigned  n_bits=16  bin_pt=0  align_bp=on  dbl_ovrd=off  block_type=logical
  Posedge2 : Subsystem
  Relational2 : xbsIndex_r4/Relational  mode=a>=b  en=off  latency=0  dbl_ovrd=off  block_type=relational
  Slot Time : xbsIndex_r4/Counter  cnt_type=Free Running  cnt_to=Inf  operation=Up  start_count=1  cnt_by_val=1  arith_type=Unsigned  n_bits=NB_CNTR_SLOT  bin_pt=0  load_pin=off  rst=on  en=on  explicit_period=off  period=1  dbl_ovrd=off  use_behavioral_HDL=off  implementation=Fabric  block_type=counter
  Slot Timer : Scope  NumInputPorts=7
      settings: YMin=-5~-5~-5~-5~-5~-5~-5  YMax=5~5~5~5~5~5~5  SaveName=ScopeData5
  Slot Done : Outport
  wires:
  Posedge2/1(Q) -> Gateway Out3/1, Slot Done/1
  Gateway Out3/1 -> Slot Timer/4
  Gateway Out1/1 -> Slot Timer/2
  Gateway Out/1 -> Slot Timer/1
  Slot Time/1 -> Gateway Out1/1, Relational2/1
  [reg_Interval_Slot] -> Relational2/2
  Logical1/1 -> Slot Time/1
  Relational2/1 -> Posedge2/1(D), Logical1/1
  Inverter/1 -> Logical1/2
  [IDLE_FOR_TXDIFS] -> Gateway Out/1, Slot Time/2, Inverter/1

== system wlan_mac_hw/TBTT ==
  note: Clear latch when target changes, on explicit reset or on global reset
  10LSB : xbsIndex_r4/Slice  nbits=10  boolean_output=off  mode=Lower Bit Location + Width  bit1=0  base1=MSB of Input  bit0=0  base0=LSB of Input  dbl_ovrd=off  block_type=slice
  22MSB : xbsIndex_r4/Slice  nbits=22  boolean_output=off  mode=Upper Bit Location + Width  bit1=0  base1=MSB of Input  bit0=0  base0=LSB of Input  dbl_ovrd=off  block_type=slice
  Concat : xbsIndex_r4/Concat  num_inputs=2  dbl_ovrd=off  block_type=concat
  Delay : xbsIndex_r4/Delay  rst=off  infoeditControl=Selection of Reset will increase slice count due to use of real FFs and instead of SRLs  en=off  latency=1  dbl_ovrd=off  reg_retiming=off  block_type=delay
  Logical1 : xbsIndex_r4/Logical  logical_function=OR  inputs=3  en=off  latency=0  precision=Full  arith_type=Unsigned  n_bits=8  bin_pt=2  align_bp=on  dbl_ovrd=off  block_type=logical
      settings: xl_area=[1 0 0 1 0 0 0]  block_version=VER_STRING_GOES_HERE
  Register : xbsIndex_r4/Register  init=0  rst=off  en=off  dbl_ovrd=off  block_type=register
  Register1 : xbsIndex_r4/Register  init=0  rst=off  en=off  dbl_ovrd=off  block_type=register
  Relational : xbsIndex_r4/Relational  mode=a>=b  en=off  latency=1  dbl_ovrd=off  block_type=relational
  Relational1 : xbsIndex_r4/Relational  mode=a!=b  en=off  latency=1  dbl_ovrd=off  block_type=relational
  S-R Latch1 : Subsystem
  tag scope: Status_TU_Target_Latch=global
  wires:
  [MAC_TIME_USEC_LSB] -> Register1/1
  22MSB/1 -> Concat/2
  [MAC_TIME_USEC_MSB] -> Register/1
  Concat/1 -> Relational/1  "Abs TUs"
  10LSB/1 -> Concat/1
  Register/1 -> 10LSB/1
  Register1/1 -> 22MSB/1
  [reg_TU_TARGET] -> Delay/1, Relational/2, Relational1/1
  Relational/1 -> S-R Latch1/1(S)
  Logical1/1 -> S-R Latch1/2(R)
  [reg_Reset_TU_Latch] -> Logical1/2
  [GLOBAL_RESET] -> Logical1/3
  S-R Latch1/1(Q) -> [Status_TU_Target_Latch]
  Delay/1 -> Relational1/2
  Relational1/1 -> Logical1/1

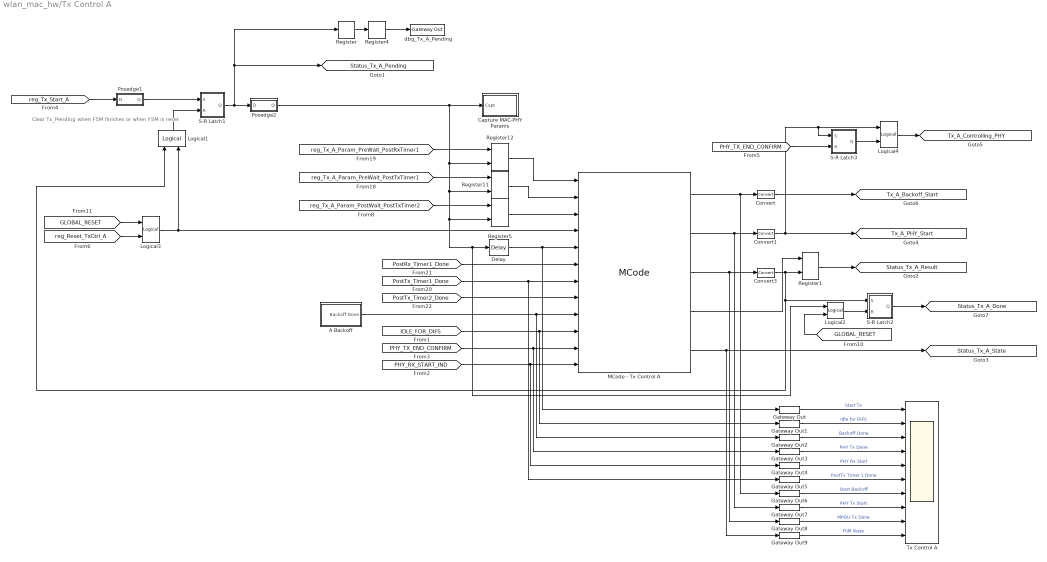
== system wlan_mac_hw/Tx Control A ==
  note: Clear Tx_Pending when FSM finishes
      | or when FSM is reset
  A Backoff : Subsystem
  Capture MAC-PHY Params : Subsystem
  Convert : xbsIndex_r4/Convert  gui_display_data_type=Boolean  arith_type=Boolean  n_bits=16  bin_pt=14  float_type=Single  exp_bits=8  fraction_bits=24  quantization=Truncate  overflow=Wrap  en=off  latency=0  dbl_ovrd=off  pipeline=off  block_type=convert
  Convert1 : xbsIndex_r4/Convert  gui_display_data_type=Boolean  arith_type=Boolean  n_bits=16  bin_pt=14  float_type=Single  exp_bits=8  fraction_bits=24  quantization=Truncate  overflow=Wrap  en=off  latency=0  dbl_ovrd=off  pipeline=off  block_type=convert
  Convert3 : xbsIndex_r4/Convert  gui_display_data_type=Boolean  arith_type=Boolean  n_bits=16  bin_pt=14  float_type=Single  exp_bits=8  fraction_bits=24  quantization=Truncate  overflow=Wrap  en=off  latency=0  dbl_ovrd=off  pipeline=off  block_type=convert
  Delay : xbsIndex_r4/Delay  rst=off  infoeditControl=Selection of Reset will increase slice count due to use of real FFs and instead of SRLs  en=off  latency=1  dbl_ovrd=off  reg_retiming=off  block_type=delay
  Gateway Out{,1..9} (10 alike) : xbsIndex_r4/Gateway Out  inherit_from_input=off  hdl_port=off  timing_constraint=None  locs_specified=off  LOCs={}  UseAsDAC=off  DACChannel='1'  block_type=gatewayout
  Logical{1..4} (4 alike) : xbsIndex_r4/Logical  logical_function=OR  inputs=2  en=off  latency=0  precision=Full  arith_type=Unsigned  n_bits=8  bin_pt=2  align_bp=on  dbl_ovrd=off  block_type=logical
      settings: xl_area=[1 0 0 1 0 0 0]  block_version=VER_STRING_GOES_HERE
  MCode - Tx Control A : xbsIndex_r4/MCode  mfname=mac_tx_ctrl_a_fsm  explicit_period=on  period=1  inputsTable={'boundInpExpr'=>['','','','','','','','','','','',''],'inputs'=>['reset','new_tx','pre_wait_postRxTimer1','pre_wait_postTxTimer1','post_wait_postTxTimer2','postRxTimer1_done','postTxTimer1_done','postTxTimer2_done','backoff_done','idle_for_difs','phy_tx_done','phy_rx_start']}  outputsTable={'outputs'=>['backoff_start','phy_tx_start','tx_done','tx_result_out','fsm_state_out'],'suppressOut'=>['off','off','off','off','off']}  dbl_ovrd=off  enable_stdout=off  enable_debug=off  suppress_output=on  defparams={}  hide_port_list={}  block_type=mcode
  Posedge1 : Subsystem
  Posedge2 : Subsystem
  Register : xbsIndex_r4/Register  init=0  rst=off  en=off  dbl_ovrd=off  block_type=register
  Register{1,5,11..12} (4 alike) : xbsIndex_r4/Register  init=0  rst=off  en=on  dbl_ovrd=off  block_type=register
  Register4 : xbsIndex_r4/Register  init=0  rst=off  en=off  dbl_ovrd=off  block_type=register
  S-R Latch1 : Subsystem
  S-R Latch2 : Subsystem
  S-R Latch3 : Subsystem
  Tx Control A : Scope  NumInputPorts=10
      settings: YMin=-5~-5~-5~-5~-5~-5~-5~-5~-5~-5  YMax=5~5~5~5~5~5~5~5~5~5
  dbg_Tx_A_Pending : xbsIndex_r4/Gateway Out  inherit_from_input=off  hdl_port=on  timing_constraint=None  locs_specified=off  LOCs={}  UseAsDAC=off  DACChannel='1'  block_type=gatewayout
  tag scope: Status_Tx_A_Done=global, Status_Tx_A_Pending=global, Status_Tx_A_Result=global, Status_Tx_A_State=global, Tx_A_Backoff_Start=global, Tx_A_Controlling_PHY=global, Tx_A_PHY_Start=global
  wires:
  [reg_Tx_Start_A] -> Posedge1/1(D)
  Posedge1/1(Q) -> S-R Latch1/1(S)
  S-R Latch1/1(Q) -> Posedge2/1(D), [Status_Tx_A_Pending], Register/1
  [reg_Tx_A_Param_PostWait_PostTxTimer2] -> Register5/1
  Delay/1 -> Gateway Out/1, MCode - Tx Control A/5
  [IDLE_FOR_DIFS] -> Gateway Out1/1, MCode - Tx Control A/10
  A Backoff/1(Backoff Done) -> Gateway Out2/1, MCode - Tx Control A/9
  [PHY_TX_END_CONFIRM] -> Gateway Out3/1, MCode - Tx Control A/11
  [PHY_RX_START_IND] -> Gateway Out4/1, MCode - Tx Control A/12
  Logical3/1 -> Logical1/2, MCode - Tx Control A/4
  MCode - Tx Control A/3 -> Convert3/1, Gateway Out8/1
  MCode - Tx Control A/2 -> Convert1/1, Gateway Out7/1
  MCode - Tx Control A/1 -> Convert/1, Gateway Out6/1
  MCode - Tx Control A/4 -> Register1/1
  Register1/1 -> [Status_Tx_A_Result]
  MCode - Tx Control A/5 -> [Status_Tx_A_State], Gateway Out9/1
  S-R Latch2/1(Q) -> [Status_Tx_A_Done]
  Convert/1 -> [Tx_A_Backoff_Start]
  Convert1/1 -> [Tx_A_PHY_Start], Logical4/1, S-R Latch3/1(S)
  Convert3/1 -> Register1/2, S-R Latch2/1(S), Logical1/1
  Logical2/1 -> S-R Latch2/2(R)
  [GLOBAL_RESET] -> Logical2/2
  Gateway Out/1 -> Tx Control A/1  "Start Tx"
  Gateway Out1/1 -> Tx Control A/2  "Idle for DIFS"
  Gateway Out2/1 -> Tx Control A/3  "Backoff Done"
  Gateway Out3/1 -> Tx Control A/4  "PHY Tx Done"
  Gateway Out4/1 -> Tx Control A/5  "PHY Rx Start"
  Gateway Out5/1 -> Tx Control A/6  "PostTx Timer 1 Done"
  Gateway Out6/1 -> Tx Control A/7  "Start Backoff"
  Gateway Out7/1 -> Tx Control A/8  "PHY Tx Start"
  Gateway Out8/1 -> Tx Control A/9  "MPDU Tx Done"
  Gateway Out9/1 -> Tx Control A/10  "FSM State"
  Register/1 -> Register4/1
  Register4/1 -> dbg_Tx_A_Pending/1
  [reg_Tx_A_Param_PreWait_PostTxTimer1] -> Register11/1
  [reg_Tx_A_Param_PreWait_PostRxTimer1] -> Register12/1
  [PostTx_Timer2_Done] -> MCode - Tx Control A/8
  [PostTx_Timer1_Done] -> Gateway Out5/1, MCode - Tx Control A/7
  [PostRx_Timer1_Done] -> MCode - Tx Control A/6
  Register5/1 -> MCode - Tx Control A/3
  Register11/1 -> MCode - Tx Control A/2
  Register12/1 -> MCode - Tx Control A/1
  [GLOBAL_RESET] -> Logical3/1
  [reg_Reset_TxCtrl_A] -> Logical3/2
  Logical1/1 -> S-R Latch1/2(R)
  Posedge2/1(Q) -> Capture MAC-PHY Params/1(Capt), Register12/2, Register11/2, Register5/2, Delay/1, Logical2/1
  S-R Latch3/1(Q) -> Logical4/2
  [PHY_TX_END_CONFIRM] -> S-R Latch3/2(R)
  Logical4/1 -> [Tx_A_Controlling_PHY]

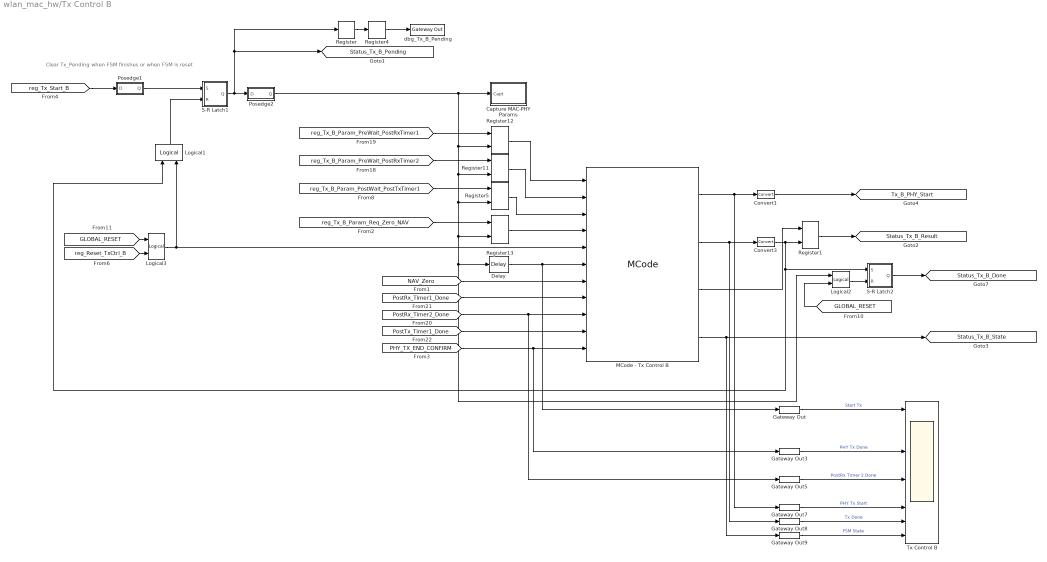
== system wlan_mac_hw/Tx Control B ==
  note: Clear Tx_Pending when FSM finishes
      | or when FSM is reset
  Capture MAC-PHY Params : Subsystem
  Convert1 : xbsIndex_r4/Convert  gui_display_data_type=Boolean  arith_type=Boolean  n_bits=16  bin_pt=14  float_type=Single  exp_bits=8  fraction_bits=24  quantization=Truncate  overflow=Wrap  en=off  latency=0  dbl_ovrd=off  pipeline=off  block_type=convert
  Convert3 : xbsIndex_r4/Convert  gui_display_data_type=Boolean  arith_type=Boolean  n_bits=16  bin_pt=14  float_type=Single  exp_bits=8  fraction_bits=24  quantization=Truncate  overflow=Wrap  en=off  latency=0  dbl_ovrd=off  pipeline=off  block_type=convert
  Delay : xbsIndex_r4/Delay  rst=off  infoeditControl=Selection of Reset will increase slice count due to use of real FFs and instead of SRLs  en=off  latency=1  dbl_ovrd=off  reg_retiming=off  block_type=delay
  Gateway Out{,3,5,7..9} (6 alike) : xbsIndex_r4/Gateway Out  inherit_from_input=off  hdl_port=off  timing_constraint=None  locs_specified=off  LOCs={}  UseAsDAC=off  DACChannel='1'  block_type=gatewayout
  Logical1 : xbsIndex_r4/Logical  logical_function=OR  inputs=2  en=off  latency=0  precision=Full  arith_type=Unsigned  n_bits=8  bin_pt=2  align_bp=on  dbl_ovrd=off  block_type=logical
      settings: xl_area=[1 0 0 1 0 0 0]  block_version=VER_STRING_GOES_HERE
  Logical2 : xbsIndex_r4/Logical  logical_function=OR  inputs=2  en=off  latency=0  precision=Full  arith_type=Unsigned  n_bits=8  bin_pt=2  align_bp=on  dbl_ovrd=off  block_type=logical
      settings: xl_area=[1 0 0 1 0 0 0]  block_version=VER_STRING_GOES_HERE
  Logical3 : xbsIndex_r4/Logical  logical_function=OR  inputs=2  en=off  latency=0  precision=Full  arith_type=Unsigned  n_bits=8  bin_pt=2  align_bp=on  dbl_ovrd=off  block_type=logical
      settings: xl_area=[1 0 0 1 0 0 0]  block_version=VER_STRING_GOES_HERE
  MCode - Tx Control B : xbsIndex_r4/MCode  mfname=mac_tx_ctrl_b_fsm  explicit_period=on  period=1  inputsTable={'boundInpExpr'=>['','','','','','','','','','',''],'inputs'=>['pre_wait_postRxTimer1','pre_wait_postRxTimer2','pre_wait_postTxTimer1','req_zero_nav','reset','new_tx','nav_zero','postRxTimer1_done','postRxTimer2_done','postTxTimer1_done','phy_tx_done']}  outputsTable={'outputs'=>['phy_tx_start','tx_done','tx_result_out','fsm_state_out'],'suppressOut'=>['off','off','off','off']}  dbl_ovrd=off  enable_stdout=off  enable_debug=off  suppress_output=on  defparams={}  hide_port_list={}  block_type=mcode
  Posedge1 : Subsystem
  Posedge2 : Subsystem
  Register : xbsIndex_r4/Register  init=0  rst=off  en=off  dbl_ovrd=off  block_type=register
  Register{1,5,11..13} (5 alike) : xbsIndex_r4/Register  init=0  rst=off  en=on  dbl_ovrd=off  block_type=register
  Register4 : xbsIndex_r4/Register  init=0  rst=off  en=off  dbl_ovrd=off  block_type=register
  S-R Latch1 : Subsystem
  S-R Latch2 : Subsystem
  Tx Control B : Scope  NumInputPorts=10
      settings: YMin=-5~-5~-5~-5~-5~-5~-5~-5~-5~-5  YMax=5~5~5~5~5~5~5~5~5~5
  dbg_Tx_B_Pending : xbsIndex_r4/Gateway Out  inherit_from_input=off  hdl_port=on  timing_constraint=None  locs_specified=off  LOCs={}  UseAsDAC=off  DACChannel='1'  block_type=gatewayout
  tag scope: Status_Tx_B_Done=global, Status_Tx_B_Pending=global, Status_Tx_B_Result=global, Status_Tx_B_State=global, Tx_B_PHY_Start=global
  wires:
  Register5/1 -> MCode - Tx Control B/3
  [PostRx_Timer1_Done] -> MCode - Tx Control B/8
  [PostRx_Timer2_Done] -> Gateway Out5/1, MCode - Tx Control B/9
  [PostTx_Timer1_Done] -> MCode - Tx Control B/10
  [reg_Tx_B_Param_PreWait_PostRxTimer1] -> Register12/1
  [reg_Tx_B_Param_PreWait_PostRxTimer2] -> Register11/1
  Register4/1 -> dbg_Tx_B_Pending/1
  Register/1 -> Register4/1
  Gateway Out9/1 -> Tx Control B/10  "FSM State"
  Gateway Out8/1 -> Tx Control B/9  "Tx Done"
  Gateway Out7/1 -> Tx Control B/8  "PHY Tx Start"
  Gateway Out5/1 -> Tx Control B/6  "PostRx Timer 2 Done"
  Gateway Out3/1 -> Tx Control B/4  "PHY Tx Done"
  Gateway Out/1 -> Tx Control B/1  "Start Tx"
  [GLOBAL_RESET] -> Logical2/2
  Logical2/1 -> S-R Latch2/2(R)
  Convert3/1 -> Register1/2, S-R Latch2/1(S), Logical1/1
  Convert1/1 -> [Tx_B_PHY_Start]
  S-R Latch2/1(Q) -> [Status_Tx_B_Done]
  MCode - Tx Control B/4 -> Gateway Out9/1, [Status_Tx_B_State]
  Register1/1 -> [Status_Tx_B_Result]
  MCode - Tx Control B/3 -> Register1/1
  MCode - Tx Control B/1 -> Gateway Out7/1, Convert1/1
  MCode - Tx Control B/2 -> Gateway Out8/1, Convert3/1
  Logical1/1 -> S-R Latch1/2(R)
  [PHY_TX_END_CONFIRM] -> Gateway Out3/1, MCode - Tx Control B/11
  Delay/1 -> Gateway Out/1, MCode - Tx Control B/6
  [reg_Tx_B_Param_PostWait_PostTxTimer1] -> Register5/1
  S-R Latch1/1(Q) -> Register/1, [Status_Tx_B_Pending], Posedge2/1(D)
  Posedge1/1(Q) -> S-R Latch1/1(S)
  [reg_Tx_Start_B] -> Posedge1/1(D)
  [NAV_Zero] -> MCode - Tx Control B/7
  Register13/1 -> MCode - Tx Control B/4
  [reg_Tx_B_Param_Req_Zero_NAV] -> Register13/1
  Register11/1 -> MCode - Tx Control B/2
  Register12/1 -> MCode - Tx Control B/1
  Logical3/1 -> MCode - Tx Control B/5, Logical1/2
  [GLOBAL_RESET] -> Logical3/1
  [reg_Reset_TxCtrl_B] -> Logical3/2
  Posedge2/1(Q) -> Capture MAC-PHY Params/1(Capt), Register12/2, Register11/2, Register5/2, Register13/2, Delay/1, Logical2/1
